simulink subsystem "PMPUnit"  (R2024b)
settings: Solver=VariableStepAuto  StartTime=0.0  StopTime=10.0  RelTol=1e-3
undefined symbols (not defined in the file): numPMPEntries
libraries: hdlsllib x4, dspstat3 x1, simulink x1
settings Model: Creator=stefano  LastModifiedBy=stefano

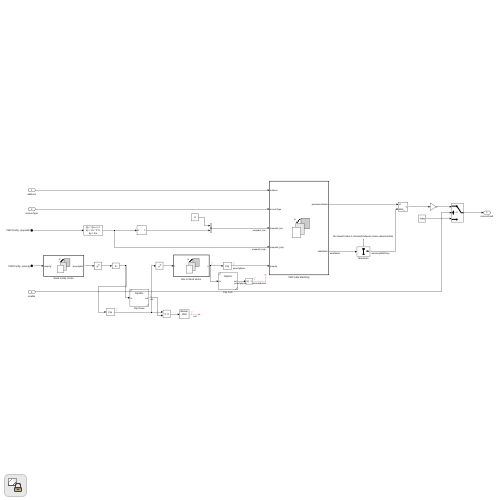
[thumbnail: Simulink's stored preview of the top-level diagram]
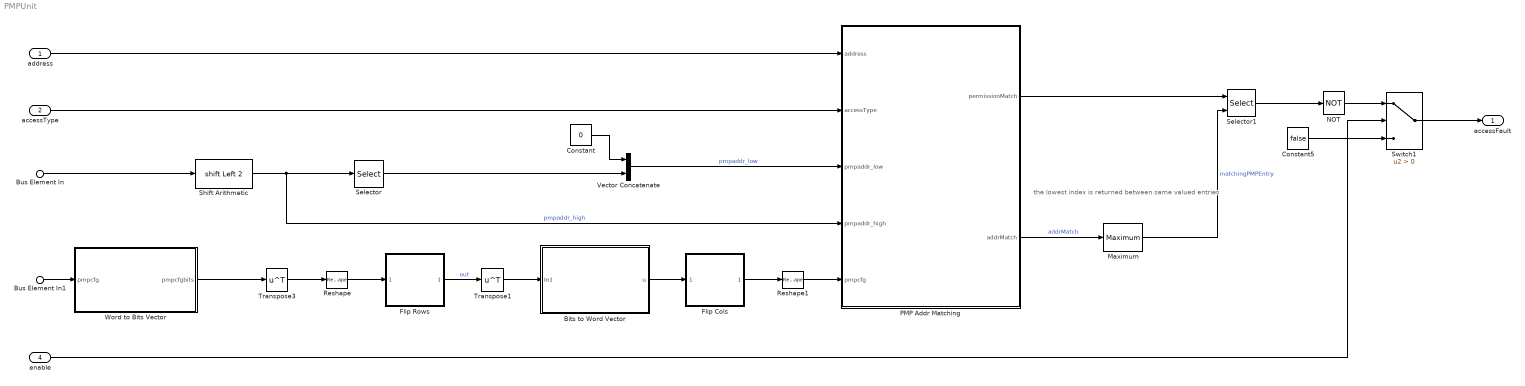
== system PMPUnit ==
  note: the lowest index is returned between same valued entries
  address : Inport
  accessType : Inport  Port=2
  Bus Element In : Inport  Port=3  PortName=PMPConfig  Element=pmpaddr
  Bus Element In1 : Inport  Port=3  PortName=PMPConfig  Element=pmpcfg
  enable : Inport  Port=4
  Bits to Word Vector : Subsystem  TreatAsAtomicUnit=on
  Constant : Constant  Value=0  OutDataTypeStr=Inherit: Inherit via back propagation  SampleTime=-1
  Constant5 : Constant  Value=false  SampleTime=-1
  Flip Cols : Subsystem  ReferencedSubsystem=FlipHDL  flipAlong=Columns
  Flip Rows : Subsystem  ReferencedSubsystem=FlipHDL  flipAlong=Rows
  Maximum : dspstat3/Maximum  operation=maximum  fcn=Index  indexBase=Zero  operateOver=Each column  Dimension=1  InputProcessing=Columns as channels (frame based)  reset=None  roiEnable=off  roiType=Rectangles  roiPortion=Entire ROI  roiOutput=Individual statistics for each ROI  roiFlag=off  roundingMode=Floor  overflowMode=off  accumDataTypeStr=Inherit: Same as product output  accumLastDataTypeStr=Inherit: Same as product output
      settings: LibrarySourceBlock=dsphdlsupportstat/Maximum
  NOT : Logic  Operator=NOT  IconShape=distinctive  AllPortsSameDT=off  OutDataTypeStr=boolean
  PMP Addr Matching : Subsystem  TreatAsAtomicUnit=on
  Reshape : Reshape  OutputDimensionality=Customize  OutputDimensions=[8, numPMPEntries]
  Reshape1 : Reshape
  Selector : Selector  InputPortWidth=numPMPEntries  IndexOptions=Index vector (dialog)  Indices=1:numPMPEntries-1  OutputSizes=1
  Selector1 : Selector  IndexMode=Zero-based  InputPortWidth=numPMPEntries  IndexOptions=Index vector (port)  Indices=[1 3]  OutputSizes=1
  Shift Arithmetic : ArithShift  BitShiftNumber=2  BitShiftDirection=Left
  Switch1 : Switch  Criteria=u2 > Threshold  SaturateOnIntegerOverflow=off  InputSameDT=off
  Transpose1 : Math  Operator=transpose
  Transpose3 : Math  Operator=transpose
  Vector Concatenate : Concatenate
  Word to Bits Vector : Subsystem  TreatAsAtomicUnit=on
  accessFault : Outport
  wires:
  Reshape1/1 -> PMP Addr Matching/5(pmpcfg)
  NOT/1 -> Switch1/1
  PMP Addr Matching/1(permissionMatch) -> Selector1/1
  Maximum/1 -> Selector1/2  "matchingPMPEntry"
  Selector1/1 -> NOT/1
  PMP Addr Matching/2(addrMatch) -> Maximum/1  "addrMatch"
  address/1 -> PMP Addr Matching/1(address)
  Constant/1 -> Vector Concatenate/1
  Selector/1 -> Vector Concatenate/2
  Vector Concatenate/1 -> PMP Addr Matching/3(pmpaddr_low)  "pmpaddr_low"
  Bus Element In1/1 -> Word to Bits Vector/1(pmpcfg)
  accessType/1 -> PMP Addr Matching/2(accessType)
  Shift Arithmetic/1 -> PMP Addr Matching/4(pmpaddr_high), Selector/1  "pmpaddr_high"
  Bus Element In/1 -> Shift Arithmetic/1
  Word to Bits Vector/1(pmpcfgbits) -> Transpose3/1
  Transpose1/1 -> Bits to Word Vector/1(In1)
  Transpose3/1 -> Reshape/1
  Flip Cols/1 -> Reshape1/1
  Constant5/1 -> Switch1/3
  Switch1/1 -> accessFault/1
  enable/1 -> Switch1/2
  Bits to Word Vector/1(u) -> Flip Cols/1
  Flip Rows/1 -> Transpose1/1  "out"
  Reshape/1 -> Flip Rows/1

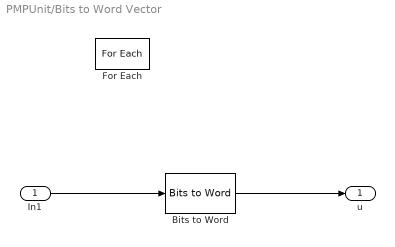
== system PMPUnit/Bits to Word Vector ==
  In1 : Inport  Partition=on  PartitionDimension=1  PartitionWidth=1  PartitionOffset=0
  Bits to Word : hdlsllib/Logic and Bit Operations/Bits to Word  bitOrder=LSB first  signedOutputValues=Unsigned
  For Each : ForEach  DisableCoverage=on
  u : Outport  ConcatenationDimension=1
  wires:
  In1/1 -> Bits to Word/1
  Bits to Word/1 -> u/1

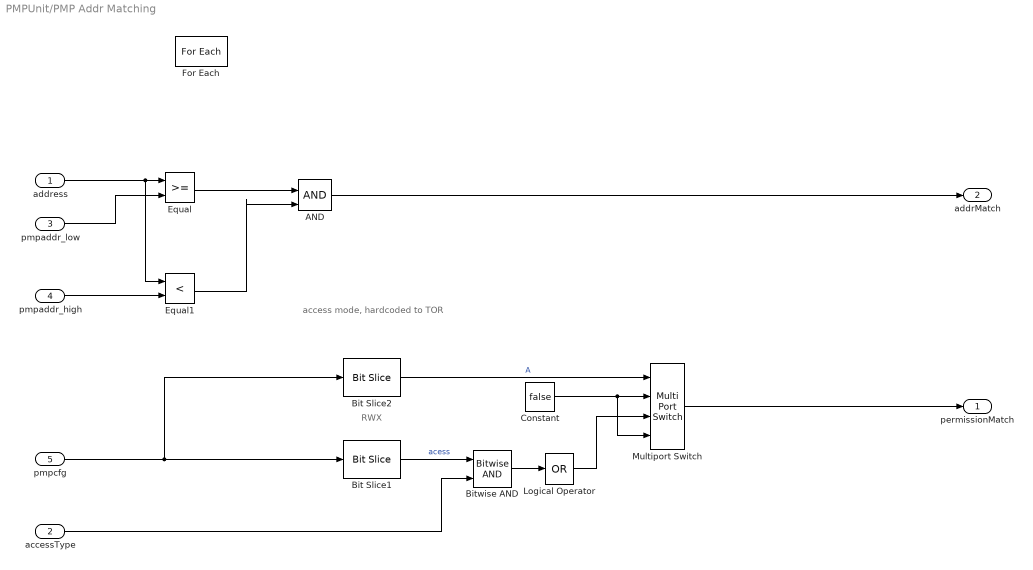
== system PMPUnit/PMP Addr Matching ==
  note: RWX
  note: access mode, hardcoded to TOR
  address : Inport
  accessType : Inport  Port=2
  pmpaddr_low : Inport  Port=3  Partition=on  PartitionDimension=1  PartitionWidth=1  PartitionOffset=0
  pmpaddr_high : Inport  Port=4  Partition=on  PartitionDimension=1  PartitionWidth=1  PartitionOffset=0
  pmpcfg : Inport  Port=5  Partition=on  PartitionDimension=1  PartitionWidth=1  PartitionOffset=0
  AND : Logic  IconShape=distinctive  AllPortsSameDT=off  OutDataTypeStr=boolean
  Bit Slice1 : hdlsllib/Logic and Bit Operations/Bit Slice  lidx=2  ridx=0
  Bit Slice2 : hdlsllib/Logic and Bit Operations/Bit Slice  lidx=4  ridx=3
  Bitwise AND : simulink/Logic and Bit Operations/Bitwise Operator  logicop=AND  UseBitMask=off  NumInputPorts=2  BitMask=bin2dec('11011001')  BitMaskRealWorld=Stored Integer
      settings: LibrarySourceBlock=|
      | simulink/Quick Insert/Logic and Bit
      | Operations/Bitwise AND
  Constant : Constant  Value=false  SampleTime=-1
  Equal : RelationalOperator  OutDataTypeStr=boolean  RndMeth=Simplest  InputSameDT=off
  Equal1 : RelationalOperator  Operator=<  OutDataTypeStr=boolean  RndMeth=Simplest  InputSameDT=off
  For Each : ForEach  DisableCoverage=on
  Logical Operator : Logic  Operator=OR  Inputs=1  AllPortsSameDT=off  OutDataTypeStr=boolean
  Multiport Switch : MultiPortSwitch  DataPortOrder=Zero-based contiguous  zeroidx=on  SaturateOnIntegerOverflow=off  InputSameDT=off
  permissionMatch : Outport  ConcatenationDimension=1
  addrMatch : Outport  Port=2  ConcatenationDimension=1
  wires:
  Logical Operator/1 -> Multiport Switch/3
  Bit Slice2/1 -> Multiport Switch/1  "A"
  Bit Slice1/1 -> Bitwise AND/1  "acess"
  pmpcfg/1 -> Bit Slice2/1, Bit Slice1/1
  address/1 -> Equal1/1, Equal/1
  pmpaddr_low/1 -> Equal/2
  pmpaddr_high/1 -> Equal1/2
  Equal/1 -> AND/1
  Equal1/1 -> AND/2
  accessType/1 -> Bitwise AND/2
  Constant/1 -> Multiport Switch/2, Multiport Switch/4
  Bitwise AND/1 -> Logical Operator/1
  Multiport Switch/1 -> permissionMatch/1
  AND/1 -> addrMatch/1

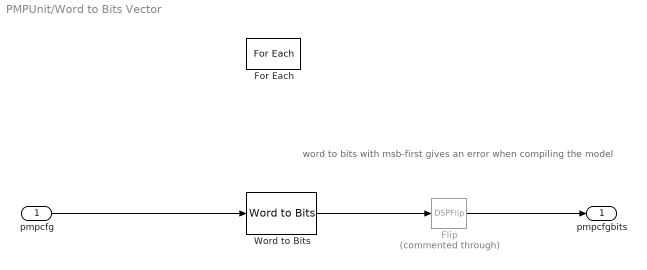
== system PMPUnit/Word to Bits Vector ==
  note: word to bits with msb-first gives an error when compiling the model
  pmpcfg : Inport  Partition=on  PartitionDimension=1  PartitionWidth=1  PartitionOffset=0
  Flip : DSPFlip  Commented=through  dim=Rows
  For Each : ForEach  DisableCoverage=on
  Word to Bits : hdlsllib/Logic and Bit Operations/Word to Bits  maxWordLength=32  bitOrder=LSB first
  pmpcfgbits : Outport  ConcatenationDimension=1
  wires:
  Flip/1 -> pmpcfgbits/1
  pmpcfg/1 -> Word to Bits/1
  Word to Bits/1 -> Flip/1
